simulink subsystem "InversePendulum"  (R2025a)
settings: Solver=VariableStepAuto  StartTime=0.0  StopTime=10.0  RelTol=1e-3
settings Model: Creator=Глеб  LastModifiedBy=Глеб

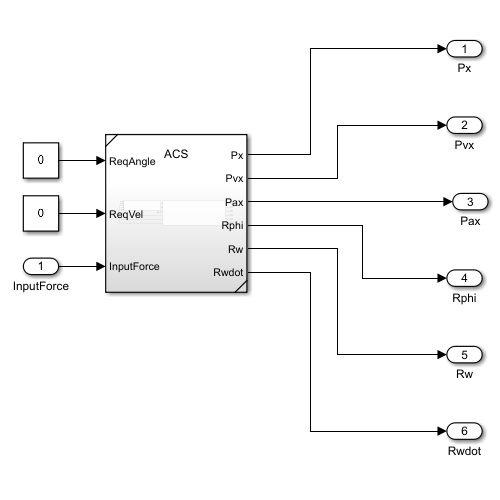
[thumbnail: Simulink's stored preview of the top-level diagram]
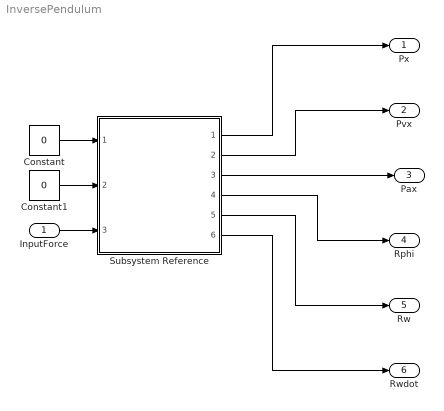
== system InversePendulum ==
  InputForce : Inport
  Constant : Constant  Value=0
  Constant1 : Constant  Value=0
  Subsystem Reference : Subsystem  ReferencedSubsystem=ACS
  Px : Outport
  Pvx : Outport  Port=2
  Pax : Outport  Port=3
  Rphi : Outport  Port=4
  Rw : Outport  Port=5
  Rwdot : Outport  Port=6
  wires:
  Subsystem Reference/1 -> Px/1
  Subsystem Reference/2 -> Pvx/1
  Subsystem Reference/6 -> Rwdot/1
  Subsystem Reference/5 -> Rw/1
  InputForce/1 -> Subsystem Reference/3
  Constant/1 -> Subsystem Reference/1
  Subsystem Reference/4 -> Rphi/1
  Subsystem Reference/3 -> Pax/1
  Constant1/1 -> Subsystem Reference/2
